simulink model "sim3"  (R2023a)
settings: Solver=VariableStepAuto  StartTime=0.0  StopTime=czas_symulacji  RelTol=1e-3
values from neighbouring files (symbols this model uses):
  cvp = vp*1.2*1000    (= 60000)    [lab3.m]
  cvw = vw*1.2*1000    (= 120000)    [lab3.m]
  dq = 0.1*qgN    (= 1000)    [lab3.m]
  dtzew = 0    [lab3.m]
  kcp = (a*qgN*(twewN-tpN))/((tpN-tzewN)*((twewN-tzewN)+a*(twewN-tpN)))    (= 19.6078431373)    [lab3.m]
  kcw = qgN/((twewN-tzewN)+a*(twewN-tpN))    (= 235.294117647)    [lab3.m]
  kcwp = a*kcw    (= 58.8235294118)    [lab3.m]
  qg0 = qgN    (= 10000)    [lab3.m]
  t0 = 1000    [lab3.m]
  tpN = 10    [lab3.m]
  twew0 = 20    [lab3.m]
  tzew0 = tzewN    (= -20)    [lab3.m]
settings Model: Creator=franc  LastModifiedBy=Boows
settings DataIOCC: ReturnWorkspaceOutputs=off
settings OptimizationCC: ReuseModelBlockBuffer=off

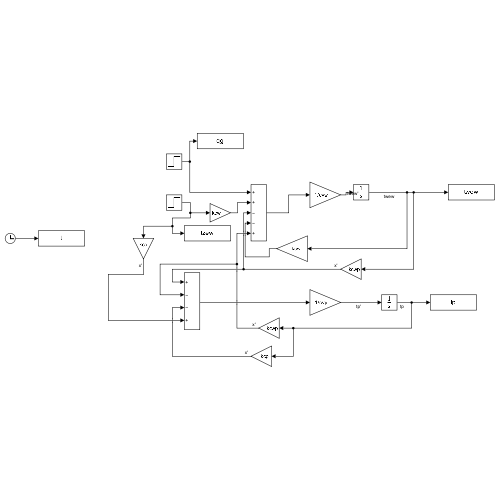
[thumbnail: Simulink's stored preview of the top-level diagram]
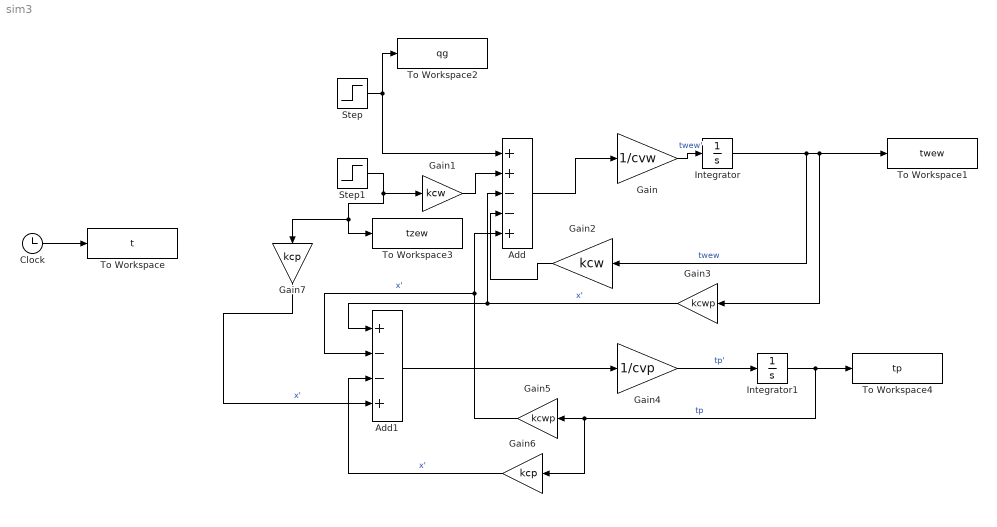
== system sim3 ==
  Add : Sum  Inputs=++--+
  Add1 : Sum  Inputs=+--+
  Clock : Clock
  Gain : Gain  Gain=1/cvw
  Gain1 : Gain  Gain=kcw
  Gain2 : Gain  Gain=kcw
  Gain3 : Gain  Gain=kcwp
  Gain4 : Gain  Gain=1/cvp
  Gain5 : Gain  Gain=kcwp
  Gain6 : Gain  Gain=kcp
  Gain7 : Gain  Gain=kcp
  Integrator : Integrator  InitialCondition=twew0
  Integrator1 : Integrator  InitialCondition=tpN
  Step : Step  Time=t0  Before=qg0  After=qg0+dq  SampleTime=0
  Step1 : Step  Time=t0  Before=tzew0  After=tzew0+dtzew  SampleTime=0
  To Workspace : ToWorkspace  VariableName=t  SaveFormat=Timeseries  SampleTime=-1
  To Workspace1 : ToWorkspace  VariableName=twew  SampleTime=-1
  To Workspace2 : ToWorkspace  VariableName=qg  SampleTime=-1
  To Workspace3 : ToWorkspace  VariableName=tzew  SampleTime=-1
  To Workspace4 : ToWorkspace  VariableName=tp  SampleTime=-1
  wires:
  Clock/1 -> To Workspace/1
  Gain/1 -> Integrator/1  "twew'"
  Integrator/1 -> Gain3/1, To Workspace1/1, Gain2/1  "twew"
  Gain2/1 -> Add/4
  Step/1 -> To Workspace2/1, Add/1
  Step1/1 -> Gain7/1, To Workspace3/1, Gain1/1
  Gain1/1 -> Add/2
  Gain3/1 -> Add1/1, Add/3  "x'"
  Integrator1/1 -> Gain6/1, Gain5/1, To Workspace4/1  "tp"
  Gain4/1 -> Integrator1/1  "tp'"
  Gain5/1 -> Add1/2, Add/5  "x'"
  Add/1 -> Gain/1
  Gain6/1 -> Add1/3  "x'"
  Gain7/1 -> Add1/4  "x'"
  Add1/1 -> Gain4/1
